simulink model "CS_SKILL_7_AM_and_FM_SPECTRUM"  (R2024a)
settings: Solver=VariableStepAuto  StartTime=0.0  StopTime=5  RelTol=1e-3
libraries: commanapbnd3 x2, dspxfrm3 x1, dspsrcs4 x1
settings Model: Creator=dev22  LastModifiedBy=dev22
settings RTWCC: GPUComputeCapability=3.5

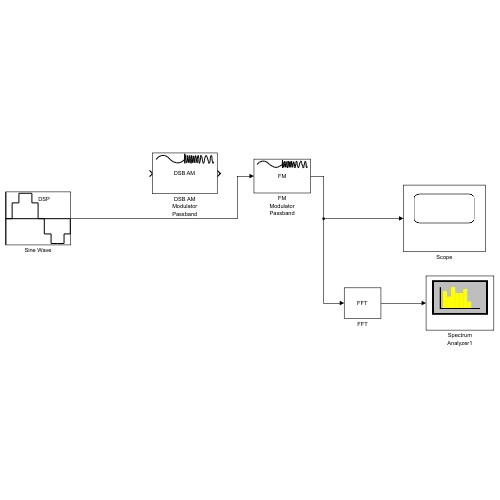
[thumbnail: Simulink's stored preview of the top-level diagram]
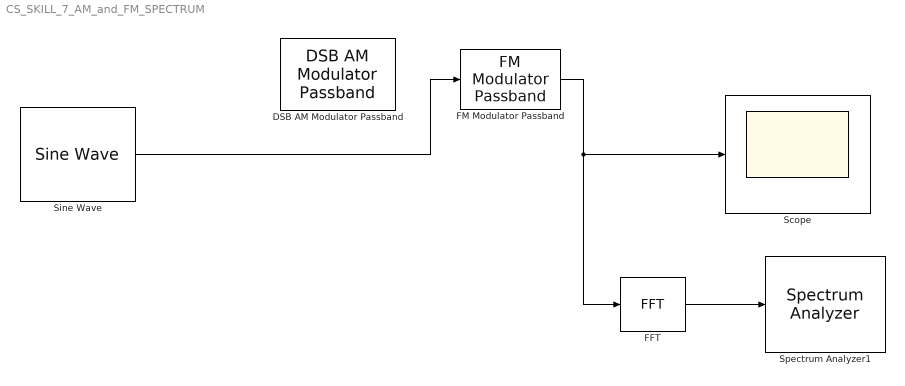
== system CS_SKILL_7_AM_and_FM_SPECTRUM ==
  DSB AM Modulator Passband : commanapbnd3/DSB AM Modulator Passband  Fc=200  Ph=0  Offset=1
  FFT : dspxfrm3/FFT  FFTImplementation=Auto  CompMethod=Table lookup  TableOpt=NEW  TableOptActive=Speed  BitRevOrder=off  Normalize=off  InheritFFTLength=on  FFTLength=64  WrapInput=on  roundingMode=Floor  overflowMode=off  firstCoeffDataTypeStr=Inherit: Same word length as input  firstCoeffLastDataTypeStr=Inherit: Same word length as input  outputMin=[]  outputMax=[]
  FM Modulator Passband : commanapbnd3/FM Modulator Passband  Fc=200  Ph=0  Kc=10
  Scope : Scope
  Sine Wave : dspsrcs4/Sine Wave  Amplitude=1  Frequency=10  Phase=0  SampleMode=Discrete  OutComplex=Real  CompMethod=Trigonometric fcn  TableSize=Speed  SampleTime=1/1000  SamplesPerFrame=1  ResetState=Restart at time zero  OutputFrames=off  dataType=double  wordLen=16  udDataType=sfix(16)  fracBitsMode=Best precision  numFracBits=15  OutDataTypeStr=double  LastOutDataTypeStr=double
  Spectrum Analyzer1 : SpectrumAnalyzer  WindowPosition=[769.000000,49.000000,766.000000,784.000000,]  ScopeFrameLocation=window  Span=1000  StartFrequency=-500  StopFrequency=500  YLimits=[-9.785635882302214,13.28885305637401]
  wires:
  FFT/1 -> Spectrum Analyzer1/1
  Sine Wave/1 -> FM Modulator Passband/1
  FM Modulator Passband/1 -> FFT/1, Scope/1
